simulink model "gm_PN_generatorV2"  (R2020a)
settings: Solver=FixedStepDiscrete  StartTime=0.0  StopTime=20  RelTol=1e-3
undefined symbols (not defined in the file or in its folder): filt
libraries: commdigbbndpm3 x2, dspmlti4 x2, commfilt2 x2, commchan3 x1, commseqgen3 x1
settings Model: Creator=juanj  LastModifiedBy=juanj
settings OptimizationCC: BlockReduction=off  ConditionallyExecuteInputs=off  DefaultParameterBehavior=Inlined
settings DebuggingCC: AlgebraicLoopMsg=error  InheritedTsInSrcMsg=none  SingleTaskRateTransMsg=error
settings HardwareCC: ProdBitPerPointer=32  ProdBitPerSizeT=32  ProdBitPerPtrDiffT=32  ProdLargestAtomicFloat=None  ProdIntDivRoundTo=Undefined  ProdEndianess=Unspecified  ProdWordSize=32  ProdHWDeviceType=ASIC/FPGA->ASIC/FPGA  TargetBitPerPointer=64  TargetBitPerSizeT=64  TargetBitPerPtrDiffT=64  TargetLongLongMode=on  TargetIntDivRoundTo=Zero  TargetEndianess=LittleEndian  TargetWordSize=64  TargetHWDeviceType=Custom Processor->MATLAB Host Computer  ProdEqTarget=off

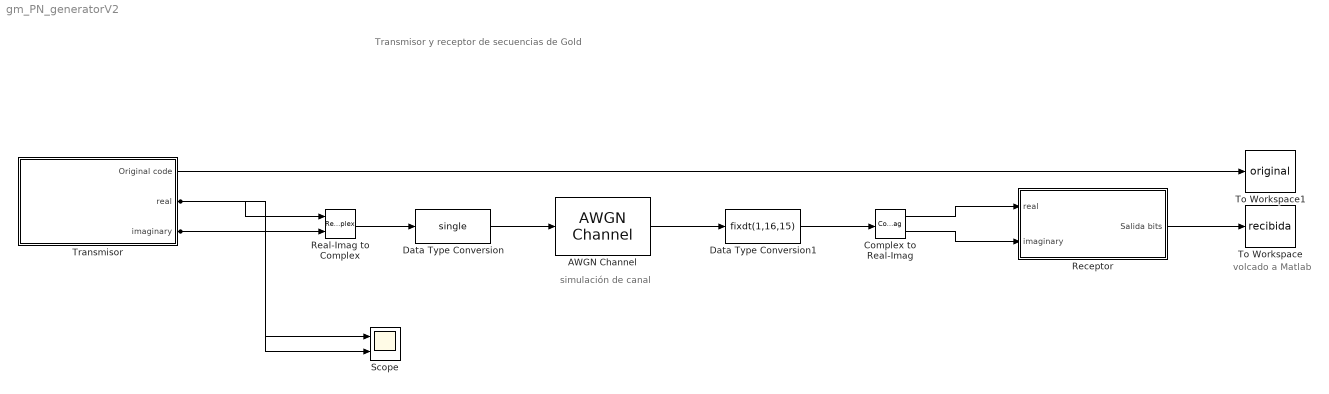
== system gm_PN_generatorV2 ==
  note: Transmisor y receptor de secuencias de Gold
  note: simulación de canal
  note: volcado a Matlab
  AWGN Channel : commchan3/AWGN Channel  InputProcessing=Columns as channels (frame based)  seed=67  noiseMode="Signal to noise ratio  (Es/No)"  EbNodB=10  EsNodB=10  SNRdB=10  bitsPerSym=1  Ps=1  Tsym=0.1  variance=1
  Complex to Real-Imag : ComplexToRealImag
  Data Type Conversion : DataTypeConversion  OutDataTypeStr=single
  Data Type Conversion1 : DataTypeConversion  OutDataTypeStr=fixdt(1,16,15)
  Real-Imag to Complex : RealImagToComplex
  Receptor : Subsystem  TreatAsAtomicUnit=on
  Scope : Scope  NumInputPorts=2
  To Workspace : ToWorkspace  VariableName=recibida  SampleTime=-1
      settings: Save2DSignal=2-D array (concatenate along first dimension)
  To Workspace1 : ToWorkspace  VariableName=original  SampleTime=-1
      settings: Save2DSignal=2-D array (concatenate along first dimension)
  Transmisor : Subsystem  TreatAsAtomicUnit=on
  wires:
  Transmisor/1(Original code) -> To Workspace1/1
  Data Type Conversion/1 -> AWGN Channel/1
  Data Type Conversion1/1 -> Complex to Real-Imag/1
  AWGN Channel/1 -> Data Type Conversion1/1
  Complex to Real-Imag/2 -> Receptor/2(imaginary)
  Complex to Real-Imag/1 -> Receptor/1(real)
  Transmisor/2(real) -> Real-Imag to Complex/1, Scope/1
  Transmisor/3(imaginary) -> Real-Imag to Complex/2, Scope/2
  Real-Imag to Complex/1 -> Data Type Conversion/1
  Receptor/1(Salida bits) -> To Workspace/1

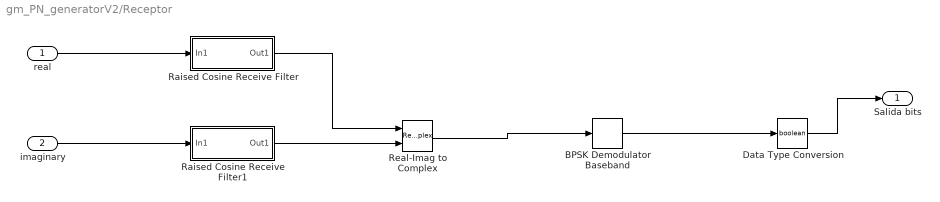
== system gm_PN_generatorV2/Receptor ==
  real : Inport  OutDataTypeStr=fixdt(1, 16, 15)  PortDimensions=1  SampleTime=0.000625
  imaginary : Inport  Port=2  OutDataTypeStr=fixdt(1, 16, 15)  PortDimensions=1  SampleTime=0.000625
  BPSK Demodulator Baseband : commdigbbndpm3/BPSK Demodulator Baseband  DecType=Hard decision  VarSource=Dialog  Variance=1  Ph=0  outDtype=Inherit via internal rule  derotateFactorWordLen=16  derotateFactorDataTypeStr=Inherit: Same word length as input  derotateFactorLastDataTypeStr=Inherit: Same word length as input
  Data Type Conversion : DataTypeConversion  OutDataTypeStr=boolean  SampleTime=0.01
  Raised Cosine Receive Filter : Subsystem  mask(Raised Cosine Receive Filter){filtType=Square root, R=double(0.5), filtSpan=double(16), N=double(16), downFactor=double(16), downOffset=double(0), filterGain=double(2), InputProcessing=Elements as channels (sample based), RateOptions=Allow multirate processing, framing=Mute, checkCoeff=off, variableName=rcRxFilt, currentFiltSpan=double(16), D=double(8), inputOffset=double(0), sampMode=Mute, saveAsFlag=double(0), rateMode=Downsampling, checkGain=Normalized, launchFVT=on, roundingMode=Floor, overflowMode=off, coeffMode=Same word length as input, coeffWordLength=double(16), coeffFracLength=double(15), coeffDataTypeStr=Inherit: Same word length as input, coeffMin=[], coeffMax=[], coeffLastDataTypeStr=Inherit: Same word length as input, prodOutputMode=Same as input, prodOutputWordLength=double(16), prodOutputFracLength=double(0), prodOutputDataTypeStr=Inherit: Same as input, prodOutputLastDataTypeStr=Inherit: Same as input, accumMode=Same as product output, accumWordLength=double(32), accumFracLength=double(30), accumDataTypeStr=Inherit: Same as product output, accumLastDataTypeStr=Inherit: Same as product output, outputMode=Same as accumulator, outputWordLength=double(16), outputFracLength=double(15), outputDataTypeStr=Inherit: Same as accumulator, outputMin=[], outputMax=[], outputLastDataTypeStr=Inherit: Same as accumulator, LockScale=off}
      mask prompts: filtType "Filter shape:"; R "Rolloff factor:"; filtSpan "Filter span in symbols:"; N "Input samples per symbol:"; downFactor "Decimation factor:"; downOffset "Decimation offset:"; filterGain "Linear amplitude filter gain:"; InputProcessing "dsp:FIRMultirateBlockDialog:InputProc_MP"; RateOptions "dsp:FIRMultirateBlockDialog:RateOptions_MP"; checkCoeff "Export filter coefficients to workspace"; variableName "Coefficient variable name:"; currentFiltSpan "Current filter span in symbols:"; D "Group delay (number of symbols):"; sampMode "Input sampling mode:"; saveAsFlag "Save_as flag:"; rateMode "Output mode:"; checkGain "Filter gain:"; launchFVT "Visualize filter with FVTool"; roundingMode "dspshared:FixptDialog:roundingMode"; overflowMode "Simulink:masks:SaturateOnIntegerOverflow_MP"; LockScale "dspshared:FixptDialog:lockAgnstChanges"
      mask help: Filter the input, and, if selected, downsample, using a normal or square root raised cosine FIR filter.
      mask init:
      | commblkrcfiltrx(gcbh,'frameupgrademultirate');
      | 
      | [filt, icon, err] = commblkrcfiltrx(gcbh,'init', ...
      |     filtType, R, filtSpan, currentFiltSpan, D, N, filterGain, ...
      |     checkCoeff, variableName, downFactor, downOffset);
      | 
      | % Set sample modes of underlying blocks
      | commblkrcfiltrx(gcb,'setFIRDecim', InputProcessing, RateOptions, ...
      |     roundingMode, overflowMode, LockScale);
      | 
      | if(~isempty(err.msg))
      | 	error(err.eID,err.msg);
      | end
      mask Help: eval('blocksethelp');
      mask TypeOptions filtType: Normal | Square root
      mask TypeOptions InputProcessing: Columns as channels (frame based) | Elements as channels (sample based)
      mask Callback InputProcessing: commblkrcfiltrx(gcbh,'cbInputProcessing');
      mask TypeOptions RateOptions: Enforce single-rate processing | Allow multirate processing
      mask TypeOptions framing: Enforce single-rate processing | Allow multirate processing | Maintain input frame rate | Maintain input frame size | Mute
      mask Callback checkCoeff: commblkrcfiltrx(gcbh,'cbCheckCoeff');
      mask Callback variableName: commblkrcfiltrx(gcbh,'dialogdynamic');
      mask TypeOptions sampMode: Frame-based | Sample-based | Mute
      mask TypeOptions rateMode: Downsampling | None
      mask TypeOptions checkGain: Normalized | User-specified
      mask TypeOptions roundingMode: Ceiling | Convergent | Floor | Nearest | Round | Simplest | Zero
      mask TypeOptions coeffMode: Same word length as input | Specify word length | Binary point scaling | Slope and bias scaling
      mask TypeOptions prodOutputMode: Same as input | Binary point scaling | Slope and bias scaling
      mask TypeOptions accumMode: Same as product output | Same as input | Binary point scaling | Slope and bias scaling
      mask TypeOptions outputMode: Same as accumulator | Same as input | Binary point scaling | Slope and bias scaling
      mask Display:
      | plot(0,0,1,1,icon.xx,icon.plot);
      | text(icon.x,icon.y,icon.str,'horiz','center');
  Raised Cosine Receive Filter1 : Subsystem  mask(Raised Cosine Receive Filter){filtType=Square root, R=double(0.5), filtSpan=double(16), N=double(16), downFactor=double(16), downOffset=double(0), filterGain=double(2), InputProcessing=Elements as channels (sample based), RateOptions=Allow multirate processing, framing=Mute, checkCoeff=off, variableName=rcRxFilt1, currentFiltSpan=double(16), D=double(8), inputOffset=double(0), sampMode=Mute, saveAsFlag=double(0), rateMode=Downsampling, checkGain=Normalized, launchFVT=on, roundingMode=Floor, overflowMode=off, coeffMode=Same word length as input, coeffWordLength=double(16), coeffFracLength=double(15), coeffDataTypeStr=Inherit: Same word length as input, coeffMin=[], coeffMax=[], coeffLastDataTypeStr=Inherit: Same word length as input, prodOutputMode=Same as input, prodOutputWordLength=double(16), prodOutputFracLength=double(0), prodOutputDataTypeStr=Inherit: Same as input, prodOutputLastDataTypeStr=Inherit: Same as input, accumMode=Same as product output, accumWordLength=double(32), accumFracLength=double(30), accumDataTypeStr=Inherit: Same as product output, accumLastDataTypeStr=Inherit: Same as product output, outputMode=Same as accumulator, outputWordLength=double(16), outputFracLength=double(15), outputDataTypeStr=Inherit: Same as accumulator, outputMin=[], outputMax=[], outputLastDataTypeStr=Inherit: Same as accumulator, LockScale=off}
      mask prompts: filtType "Filter shape:"; R "Rolloff factor:"; filtSpan "Filter span in symbols:"; N "Input samples per symbol:"; downFactor "Decimation factor:"; downOffset "Decimation offset:"; filterGain "Linear amplitude filter gain:"; InputProcessing "dsp:FIRMultirateBlockDialog:InputProc_MP"; RateOptions "dsp:FIRMultirateBlockDialog:RateOptions_MP"; checkCoeff "Export filter coefficients to workspace"; variableName "Coefficient variable name:"; currentFiltSpan "Current filter span in symbols:"; D "Group delay (number of symbols):"; sampMode "Input sampling mode:"; saveAsFlag "Save_as flag:"; rateMode "Output mode:"; checkGain "Filter gain:"; launchFVT "Visualize filter with FVTool"; roundingMode "dspshared:FixptDialog:roundingMode"; overflowMode "Simulink:masks:SaturateOnIntegerOverflow_MP"; LockScale "dspshared:FixptDialog:lockAgnstChanges"
      mask help: Filter the input, and, if selected, downsample, using a normal or square root raised cosine FIR filter.
      mask init: same as gm_PN_generatorV2/Receptor/Raised Cosine Receive Filter
      mask Help: eval('blocksethelp');
      mask TypeOptions filtType: Normal | Square root
      mask TypeOptions InputProcessing: Columns as channels (frame based) | Elements as channels (sample based)
      mask Callback InputProcessing: commblkrcfiltrx(gcbh,'cbInputProcessing');
      mask TypeOptions RateOptions: Enforce single-rate processing | Allow multirate processing
      mask TypeOptions framing: Enforce single-rate processing | Allow multirate processing | Maintain input frame rate | Maintain input frame size | Mute
      mask Callback checkCoeff: commblkrcfiltrx(gcbh,'cbCheckCoeff');
      mask Callback variableName: commblkrcfiltrx(gcbh,'dialogdynamic');
      mask TypeOptions sampMode: Frame-based | Sample-based | Mute
      mask TypeOptions rateMode: Downsampling | None
      mask TypeOptions checkGain: Normalized | User-specified
      mask TypeOptions roundingMode: Ceiling | Convergent | Floor | Nearest | Round | Simplest | Zero
      mask TypeOptions coeffMode: Same word length as input | Specify word length | Binary point scaling | Slope and bias scaling
      mask TypeOptions prodOutputMode: Same as input | Binary point scaling | Slope and bias scaling
      mask TypeOptions accumMode: Same as product output | Same as input | Binary point scaling | Slope and bias scaling
      mask TypeOptions outputMode: Same as accumulator | Same as input | Binary point scaling | Slope and bias scaling
      mask Display:
      | plot(0,0,1,1,icon.xx,icon.plot);
      | text(icon.x,icon.y,icon.str,'horiz','center');
  Real-Imag to Complex : RealImagToComplex  ConstantPart="fi(0,1,16,15,\"hex\",\"0000\")"  SampleTime=0.01
  Salida bits : Outport
  wires:
  real/1 -> Raised Cosine Receive Filter/1(In1)
  imaginary/1 -> Raised Cosine Receive Filter1/1(In1)
  BPSK Demodulator Baseband/1 -> Data Type Conversion/1
  Data Type Conversion/1 -> Salida bits/1
  Raised Cosine Receive Filter/1(Out1) -> Real-Imag to Complex/1
  Raised Cosine Receive Filter1/1(Out1) -> Real-Imag to Complex/2
  Real-Imag to Complex/1 -> BPSK Demodulator Baseband/1

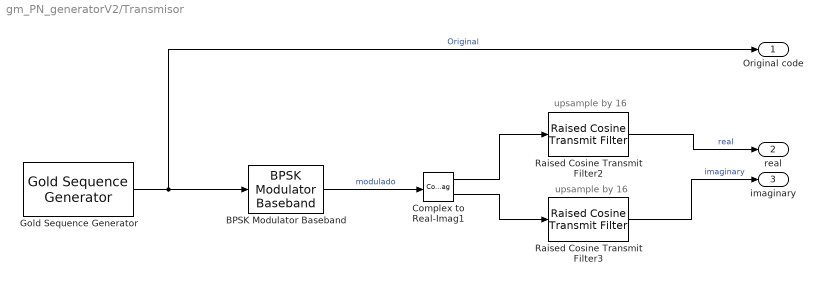
== system gm_PN_generatorV2/Transmisor ==
  note: upsample by 16
  note: upsample by 16
  BPSK Modulator Baseband : commdigbbndpm3/BPSK Modulator Baseband  Ph=0  outDtype=Fixed-point  outWordLen=16  outUDDataType=sfix(16)  outFracLenMode=Best precision  outFracLen=15  outDataTypeStr=fixdt(1,16)  outLastDataTypeStr=fixdt(1,16)
  Complex to Real-Imag1 : ComplexToRealImag
  Gold Sequence Generator : commseqgen3/Gold Sequence Generator  genPoly1='z^6 + z + 1'  iniState1=[0 1 0 1 0 1]  genPoly2='z^6 + z^5 + z^2 + z + 1'  iniState2=[0 0 0 0 0 1]  index=0  shift=0  outVarSiz=off  maxOutSizeMode=Dialog parameter  maxOutSize=[10 1]  Ts=1/100  sampPerFrame=1  reset=off  outDataType=boolean
      settings: SourceProductBaseCode=CM
  Raised Cosine Transmit Filter2 : commfilt2/Raised Cosine Transmit Filter  filtType=Square root  R=0.5  filtSpan=16  N=16  filterGain=2  RateOptions=Allow multirate processing  framing=Mute  checkCoeff=off  variableName=rcTxFilt2  checkGain=Normalized  sampMode=Mute  saveAsFlag=0  currentFiltSpan=16  D=(16)/2  launchFVT=on  roundingMode=Floor  overflowMode=off  coeffDataTypeStr=Inherit: Same word length as input  coeffMin=[]  coeffMax=[]  coeffLastDataTypeStr=Inherit: Same word length as input  outputMin=[]  outputMax=[]
  Raised Cosine Transmit Filter3 : commfilt2/Raised Cosine Transmit Filter  filtType=Square root  R=0.5  filtSpan=16  N=16  filterGain=2  RateOptions=Allow multirate processing  framing=Mute  checkCoeff=off  variableName=rcTxFilt3  checkGain=Normalized  sampMode=Mute  saveAsFlag=0  currentFiltSpan=16  D=(16)/2  launchFVT=on  roundingMode=Floor  overflowMode=off  coeffDataTypeStr=Inherit: Same word length as input  coeffMin=[]  coeffMax=[]  coeffLastDataTypeStr=Inherit: Same word length as input  outputMin=[]  outputMax=[]
  Original code : Outport
  real : Outport  Port=2
  imaginary : Outport  Port=3
  wires:
  Raised Cosine Transmit Filter2/1 -> real/1  "real"
  Complex to Real-Imag1/2 -> Raised Cosine Transmit Filter3/1
  BPSK Modulator Baseband/1 -> Complex to Real-Imag1/1  "modulado"
  Complex to Real-Imag1/1 -> Raised Cosine Transmit Filter2/1
  Gold Sequence Generator/1 -> BPSK Modulator Baseband/1, Original code/1  "Original"
  Raised Cosine Transmit Filter3/1 -> imaginary/1  "imaginary"

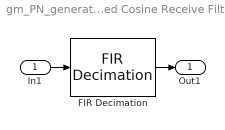
== system gm_PN_generatorV2/Receptor/Raised Cosine Receive Filter ==
  In1 : Inport  OutDataTypeStr=fixdt(1, 16, 15)  SampleTime=0.000625
  FIR Decimation : dspmlti4/FIR Decimation  FilterSource=Dialog parameters  h=filt.coeff  D=filt.decimFactor  filtStruct=Direct form  FilterObject=Hm_firdecim  framing=Allow multirate processing  inputOffset=(filt.decimFactor-filt.decimOffset)  outputBufInitCond=0  roundingMode=Floor  overflowMode=off  firstCoeffDataTypeStr=Inherit: Same word length as input  firstCoeffMin=[]  firstCoeffMax=[]  firstCoeffLastDataTypeStr=Inherit: Same word length as input  accumDataTypeStr=Inherit: Same as product output  accumLastDataTypeStr=Inherit: Same as product output  outputDataTypeStr=Inherit: Same as accumulator  outputMin=[]  outputMax=[]  outputLastDataTypeStr=Inherit: Same as accumulator
  Out1 : Outport
  wires:
  In1/1 -> FIR Decimation/1
  FIR Decimation/1 -> Out1/1

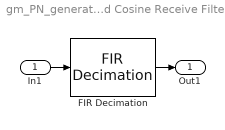
== system gm_PN_generatorV2/Receptor/Raised Cosine Receive Filter1 ==
  In1 : Inport  OutDataTypeStr=fixdt(1, 16, 15)  SampleTime=0.000625
  FIR Decimation : dspmlti4/FIR Decimation  FilterSource=Dialog parameters  h=filt.coeff  D=filt.decimFactor  filtStruct=Direct form  FilterObject=Hm_firdecim  framing=Allow multirate processing  inputOffset=(filt.decimFactor-filt.decimOffset)  outputBufInitCond=0  roundingMode=Floor  overflowMode=off  firstCoeffDataTypeStr=Inherit: Same word length as input  firstCoeffMin=[]  firstCoeffMax=[]  firstCoeffLastDataTypeStr=Inherit: Same word length as input  accumDataTypeStr=Inherit: Same as product output  accumLastDataTypeStr=Inherit: Same as product output  outputDataTypeStr=Inherit: Same as accumulator  outputMin=[]  outputMax=[]  outputLastDataTypeStr=Inherit: Same as accumulator
  Out1 : Outport
  wires:
  In1/1 -> FIR Decimation/1
  FIR Decimation/1 -> Out1/1
